simulink model "controller_v13"  (R2020b)
settings: Solver=ode4  StartTime=0.0  StopTime=inf  RelTol=1e-3
undefined symbols (not defined in the file): ctr, DiscIntNeverNeededParam, flt, IO397, mdl, rbt, rsim, som, ukf_P0_flat, ukf_prediction_time, ukf_s0, ukf_sys, ukf_use_prediction
libraries: simulink x31, slrealtimeloglib x5, slrealtimeseriallib x5, speedgoatlib_fpga_analog_io x4, slrealtimetgmanagement x3, speedgoatlib_fpga x2, speedgoatlib_fpga_dio x1, slrealtimeutilitieslib x1
(part 5 of 5)

== matlab function controller_v13/Adaptive Controller/Attitude and thrust learned NMPC/Geometric Attitude Controller ==
  data: cmd_B_torque output; R input; Omega input size=3; Rd input; Omegad input size=3; Omegadd input; tau_ext input size=3; traj_time input; ctr parameter; rbt parameter; mdl parameter; M_e_att output; M_e_angv output; M_e_cross output; M_e_ang_acc output; M_e_ext_tau output
function [cmd_B_torque, M_e_att, M_e_angv, M_e_cross, M_e_ang_acc, M_e_ext_tau]   = fcn(R, Omega, Rd, Omegad, Omegadd, tau_ext, traj_time, ctr, rbt, mdl)
%#codegen
% r: curr pos
% r_dot: curr vel
% R: current attitude
% Omega: current body rates
% rd : des pos
% rd_d: des vel
% Rd: desired attitude (rotation matrix)
% Omegad: desired angular velocity


% current attitude
R = unflatten_rotm(R);     % transform vector in rotation matrix
Omega = Omega(:);
Omegad = Omegad(:);
if ctr.rtnmpc.set_cmd_omega_y_to_zero
    Omegad(2) = 0.0;
end
%Omegad = zeros(3,1);
tau_ext = tau_ext(:);

% desired attitude & angvel
Rd = unflatten_rotm(Rd);
% inertial frame 3-axis


% thrust magnitude control, eq 19
% A = -ctr.lee.pos.kx*ex - ctr.lee.pos.kv*ev - rbt.m*mdl.g*e3; % + P.mass*xd_2dot;
% cmd_B_acc_z = dot(-A, R*e3)/rbt.m;

% Rd = get_desired_attitude_x_axis(Rd, R);
% Rd = get_desired_attitude_y_axis(Rd, R);

% inertia matrix
J = diag([ctr.lee.ixx, ctr.lee.iyy, ctr.lee.izz]);

% attitude and angular velocity errors
eR     = (1/2)*vee(Rd.'*R - R.'*Rd);
eOmega = Omega - R.'*Rd*Omegad;

% desired torque
M = zeros(3,1);
M_e_att = -ctr.lee.kR*eR;
M_e_angv = - ctr.lee.kOmega*eOmega;
M_e_cross = cross(Omega, J*Omega);
M_e_ang_acc = - J*(hat(Omega)*R'*Rd*Omegad); % TODO: ANDREA: WHY THIS IS WRONG?
if ctr.lee.ang_acc_ff
    M_e_ang_acc = M_e_ang_acc + J*Omegadd;
end
M_e_ext_tau = - [tau_ext(1); tau_ext(2); 0.0];

% reduce torqe on y after flip
if traj_time > 1.3
    M_e_ext_tau(2) = 0.1*M_e_ext_tau(2); 
end

M = M_e_att + M_e_angv + M_e_cross + M_e_ang_acc + M_e_ext_tau;
M(3) = 0.0;

att_e = eR;
cmd_B_torque = M(:);
u_lim = [ctr.rtmpc.lim.torque_x; ctr.rtmpc.lim.torque_y; ctr.rtmpc.lim.torque_z;];
cmd_B_torque = max(min(cmd_B_torque, u_lim), -u_lim);

end

function vec = vee(ss)
% function vec = vee(skewsymmetric)
%   The vee function maps a skew-symmetric 
%   matrix to a vector

% https://github.com/justinthomas/MATLAB-tools/blob/master/vee.m

if isa(ss,'sym')
    ss = expand(simplify(ss));
end

switch numel(ss)
    
    case 4
        
        if ~isequal(ss(1,2), -ss(2,1))
            disp('The provided matrix is not skew symmetric')
        end
        
        vec = ss(1,2);

    case 9

        if ~isequal(ss(3,2),-ss(2,3)) || ~isequal(ss(1,3),-ss(3,1)) || ~isequal(ss(2,1),-ss(1,2))
            disp('The provided matrix is not skew symmetric.')
            %print(ss)
        end

        vec = [ss(3,2); ss(1,3); ss(2,1)];
end

if isa(ss,'sym')
    vec = simplify(vec);
end

end

function ss = hat(vec)
% function ss = hat(vec)
%   The hat function maps a vector in R^3 (or R^1) to its
%   skew symmetric matrix in R^(3x3) (or R^(2x2))

% https://github.com/justinthomas/MATLAB-tools/blob/master/hat.m

switch length(vec)
    
    case 3
        ss = [...
            0, -vec(3), vec(2);...
            vec(3), 0, -vec(1);...
            -vec(2), vec(1), 0];
        
    case 1
        ss = [...
            0, vec; ...
            -vec, 0];
end

end

function Rd = get_desired_attitude_x_axis(Rd, R)

    e3 = [0;0;1];
    % normalized feedback function, eq 23
    b3c = Rd*e3;
    
    % Desired x axis -- current x axis
    b1d = R(:, 1);
    
    % Construct b1c, eq 38
    C = cross(b3c, b1d); % arXiv:1003.2005v3, eq ~97
    b1c = -(1/norm(C))*cross(b3c, C);
    
    b2c = C/norm(C);
    
    % computed attitude, eq 22
    Rd = [b1c b2c b3c];

end

function Rd = get_desired_attitude_y_axis(Rd, R)

    e3 = [0;0;1];
    % normalized feedback function, eq 23
    b3c = Rd*e3;
    
    % Desired y axis -- current x axis
    b2d = R(:, 2);
    
    % Construct b2c, eq 38
    C = cross(b3c, b2d); % arXiv:1003.2005v3, eq ~97
    b2c = -(1/norm(C))*cross(b3c, C);
    
    b1c = C/norm(C);
    
    % computed attitude, eq 22
    Rd = [b1c b2c b3c];

end

== matlab function controller_v13/Adaptive Controller/ground truth/Rotm2rpy1 ==
  data: R input; rpy output size=3
function rpy   = fcn(R)
    R = unflatten_rotm(R);
    ypr = rotm2eul(R); 
    rpy = [ypr(3); ypr(2); ypr(1)];
end

== matlab function controller_v13/Adaptive Controller/correct force ==
  data: Force input; corrected_force output; rbt parameter
function corrected_force = fcn(Force,rbt)
Force_error_Gs = polyval(rbt.thrust_error_poly_fit, (Force/rbt.m/9.81-1.0));
corrected_force = (Force_error_Gs)*rbt.m*9.81 + Force;
end

== matlab function controller_v13/Measurement manager/safety check system/landing condition/landing_cond ==
  data: alt input; en output; time_cond input; ctr parameter
function en = fcn(alt,time_cond,ctr)
%#codegen
if ( (time_cond<0) | (alt>ctr.landing.height) )
    en = 1;
else
    en = 0;
end
en=1;
end
% this lands the robot if the flight time is more than mdl.i_delay+2 and
% the robot is still on the ground.
